simulink model "estimator_designs_main"  (R2022b)
settings: Solver=ode4  StartTime=0.0  StopTime=T  FixedStep=0.002  RelTol=1e-3
values from neighbouring files (symbols this model uses):
  c_lat_f = u(11)    [modelBasedSpeedEstForKalman.m]    (also in validation.m = 140000)
  c_lat_r = u(12)    [modelBasedSpeedEstForKalman.m]    (also in validation.m = 150000)
  c_lon_f = u(9)    [modelBasedSpeedEstForKalman.m]    (also in validation.m = 180000)
  c_lon_r = u(10)    [modelBasedSpeedEstForKalman.m]    (also in validation.m = 200000)
  dt = u(4)    [kinematicVelocity.m]    (also in modelBasedSpeedEstForKalman.m = u(27); validation.m = 0.01)
  eps_bw_acc = 0.1    [validation.m]
  eps_ekf_m_bw_v_u = 0.5    [validation.m]
  eps_m_v = 1    [validation.m]
  m = u(7)    [modelBasedSpeedEstForKalman.m]    (also in validation.m = 3020)
  num_of_signals = 12    [validation.m]
  P0 = diag([1e-5, 1e-5, 1e-5])    [validation.m]
  Q_ekf_1 = diag([1e-5, 1e-2, 1e-2])    [validation.m]
  R = u(9)    [bestWheelSpeedUpdate.m]    (also in modelBasedSpeedEstForKalman.m = u(13); validation.m = 0.3615)
  r_COG_FL = u(10:12)    [bestWheelSpeedUpdate.m]    (also in validation.m = [wheelbase_COG_front; front_track_width / 2; 0])
  r_COG_FR = u(13:15)    [bestWheelSpeedUpdate.m]    (also in validation.m = [wheelbase_COG_front; -front_track_width / 2; 0])
  r_COG_RL = u(16:18)    [bestWheelSpeedUpdate.m]    (also in validation.m = [-wheelbase_COG_rear; rear_track_width / 2; 0])
  r_COG_RR = u(19:21)    [bestWheelSpeedUpdate.m]    (also in validation.m = [-wheelbase_COG_rear; -rear_track_width / 2; 0])
  R_ekf_1 = 1e-2    (= 0.01)    [validation.m]
  sequence_length = 50    [validation.m]
  theta_z = 7145    [validation.m]
  thr_ekf_m_bw_v_u = 5    [validation.m]
  x0 = [0.0001; 0.0001; 0.0001]    [validation.m]
undefined symbols (not defined in the file or in its folder): Discrete, Time
libraries: deeplib x2, ctrlSharedLib x1
(part 2 of 2)

== matlab function estimator_designs_main/v_u_estimators/ekf_model_bw/ekf_custom/ekf_model ==
  data: x_in input; P_in input; z_in input; Q_in input; R_in input; u_in input; fdStep input; x_out output; gateNIS input; P_out output; K_out output; nu_out output; S_out output; x_pred_out output; P_pred_out output; z_pred_out output; F_out output; H_out output; NIS_out output; status_out output
function [x_out,P_out,K_out,nu_out,S_out, ...
          x_pred_out,P_pred_out,z_pred_out, ...
          F_out,H_out,NIS_out,status_out] = ...
    ekf_modelBased_textbook_step(x_in,P_in,z_in,Q_in,R_in,u_in,fdStep,gateNIS)
% -------------------------------------------------------------------------
% Textbook EKF (single step) for state x = [v_x; v_y; w_z].
% Hard-coded:
%   Process model:    x_pred = modelBasedSpeedEstForKalman(x_in, u_in)
%   Measurement:      z = simpleMeasUpdate(x, u) = x(1)  (longitudinal speed)
%
% Inputs:
%   x_in    : 3x1 prior state estimate (k|k)
%   P_in    : 3x3 prior covariance     (k|k)
%   z_in    : scalar measurement (v_x at time k+1)
%   Q_in    : 3x3 process noise covariance (per step)
%   R_in    : scalar measurement variance
%   u_in    : NUx1 input vector for modelBasedSpeedEstForKalman (fixed size; fill ALL entries)
%   fdStep  : finite-difference step for Jacobian (e.g. 1e-5)
%   gateNIS : gating threshold (Inf to disable; e.g. 6.63 for 99% scalar)
%
% Outputs:
%   x_out       : 3x1 posterior state (k+1|k+1)
%   P_out       : 3x3 posterior covariance
%   K_out       : 3x1 Kalman gain
%   nu_out      : innovation (z - z_pred)
%   S_out       : innovation variance
%   x_pred_out  : 3x1 predicted state (k+1|k)
%   P_pred_out  : 3x3 predicted covariance
%   z_pred_out  : scalar predicted measurement
%   F_out       : 3x3 process Jacobian (finite difference)
%   H_out       : 1x3 measurement Jacobian ([1 0 0])
%   NIS_out     : normalized innovation squared (nu^2 / S)
%   status_out  : diagnostic code:
%                 0 OK
%                 1 Process model produced NaN/Inf
%                 2 FD Jacobian produced NaN/Inf (fallback F=I)
%                 3 Innovation variance invalid (S<=0 -> jittered)
%                 4 Update gated (NIS > gateNIS)
%
% Textbook equations:
%   Predict:  x^- = f(x,u);  P^- = F P F' + Q
%   z^- = h(x^-); nu = z - z^-
%   S  = H P^- H' + R
%   K  = P^- H' / S
%   x  = x^- + K nu
%   P  = (I - K H) P^- (I - K H)' + K R K'
%
% -------------------------------------------------------------------------

% ---------- Initialize outputs for safety ----------
x_out       = x_in;
P_out       = P_in;
K_out       = zeros(3,1);
nu_out      = 0;
S_out       = 1;
x_pred_out  = x_in;
P_pred_out  = P_in;
z_pred_out  = x_in(1);
F_out       = eye(3);
H_out       = [1 0 0];
NIS_out     = 0;
status_out  = 0;   % assume OK

% ---------- 1. Prediction ----------
x_pred = modelBasedSpeedEstForKalman(x_in, u_in);
if any(~isfinite(x_pred))
    status_out = 1;  % process model failure
    return;
end

% ---------- 2. Finite-difference Jacobian F = df/dx ----------
h = fdStep;
F = zeros(3,3);

% Column 1
xp = x_in; xm = x_in;
xp(1) = xp(1) + h; xm(1) = xm(1) - h;
fp = modelBasedSpeedEstForKalman(xp, u_in);
fm = modelBasedSpeedEstForKalman(xm, u_in);
if any(~isfinite(fp)) || any(~isfinite(fm))
    status_out = 2;
    F = eye(3);
else
    F(:,1) = (fp - fm)/(2*h);
end

% Column 2
xp = x_in; xm = x_in;
xp(2) = xp(2) + h; xm(2) = xm(2) - h;
fp = modelBasedSpeedEstForKalman(xp, u_in);
fm = modelBasedSpeedEstForKalman(xm, u_in);
if any(~isfinite(fp)) || any(~isfinite(fm))
    status_out = 2;
    F(:,2) = 0;  % leave existing or zero
else
    F(:,2) = (fp - fm)/(2*h);
end

% Column 3
xp = x_in; xm = x_in;
xp(3) = xp(3) + h; xm(3) = xm(3) - h;
fp = modelBasedSpeedEstForKalman(xp, u_in);
fm = modelBasedSpeedEstForKalman(xm, u_in);
if any(~isfinite(fp)) || any(~isfinite(fm))
    status_out = 2;
    F(:,3) = 0;
else
    F(:,3) = (fp - fm)/(2*h);
end

F_out = F;

% ---------- 3. Covariance prediction ----------
P_pred = F*P_in*F' + Q_in;
if any(~isfinite(P_pred(:)))
    status_out = max(status_out,2);
    P_pred = P_in + Q_in;  % simple fallback
end

% ---------- 4. Measurement prediction h(x)=x(1) ----------
z_pred = x_pred(1);
H = [1 0 0];

% ---------- 5. Innovation ----------
nu = z_in - z_pred;

% ---------- 6. Innovation variance ----------
S = P_pred(1,1) + R_in;
if ~isfinite(S) || S <= 0
    S = max(R_in,1e-9);
    status_out = max(status_out,3);
end

% ---------- 7. Kalman Gain ----------
K = P_pred(:,1) / S;

% ---------- 8. NIS ----------
NIS = (nu*nu)/S;

% ---------- 9. Gating ----------
gated = false;
if NIS > gateNIS
    x_post = x_pred;
    P_post = P_pred;
    K(:)   = 0;
    gated  = true;
    status_out = 4;
else
    % ---------- 10. Update ----------
    x_post = x_pred + K*nu;

    % ---------- 11. Covariance update (Joseph) ----------
    I = eye(3);
    IKH = I - K*H;
    P_post = IKH * P_pred * IKH' + K*R_in*K';
end

% ---------- 12. Symmetrize ----------
P_post = 0.5*(P_post + P_post');
if any(~isfinite(P_post(:)))
    status_out = max(status_out,3);
    x_post = x_in;
    P_post = P_in;
    K(:) = 0;
end

% ---------- 13. Assign outputs ----------
x_out       = x_post;
P_out       = P_post;
K_out       = K;
nu_out      = nu;
S_out       = S;
x_pred_out  = x_pred;
P_pred_out  = P_pred;
z_pred_out  = z_pred;
H_out       = H;
NIS_out     = NIS;

end

== matlab function estimator_designs_main/meas_inputs/sequence_generator/MATLAB Function1 ==
  data: SENS_IN_ai input; SENS_IN_ai_seq output; SENS_IN_ai_seq_prev input
function SENS_IN_ai_seq = sequence_generator_t(SENS_IN_ai, SENS_IN_ai_seq_prev)
% This function returns a sequence of data that will be fed into the RNN
% model

    SENS_IN_ai_seq = [SENS_IN_ai_seq_prev(:, 2 : end), SENS_IN_ai];

end

== matlab function estimator_designs_main/v_u_estimators/kf_sm_bw/meas_update_bw/best_wheel_speed_est ==
  data: u input size=23; v_u_bw output size=1; sign_acc output size=1
function [v_u_bw, sign_acc]= bestWheelSpeedUpdate(u)

omega_w_FL = u(1);
omega_w_FR = u(2);
omega_w_RL = u(3);
omega_w_RR = u(4);

delta_FL = u(5);
delta_FR = u(5);
delta_RL = u(6);
delta_RR = u(6);

w_z = u(7);

acc = u(8);

R = u(9);
r_COG_FL = u(10:12);
r_COG_FR = u(13:15);
r_COG_RL = u(16:18);
r_COG_RR = u(19:21);

eps_bw_acc = u(22);

prev_sign_acc = u(23);

w = [0; 0; w_z];

% calculating the velocities of the wheels from the wheel rotational speeds
v_w_FL = [omega_w_FL * R; 0; 0];
v_w_FR = [omega_w_FR * R; 0; 0];
v_w_RL = [omega_w_RL * R; 0; 0];
v_w_RR = [omega_w_RR * R; 0; 0];

% transforming the wheel velocities to the coordinate system in the wheels
% parallel to the one in COG
T_FL = [cos(-delta_FL), sin(-delta_FL), 0; -sin(-delta_FL), cos(-delta_FL), 0; 0, 0, 1];
T_FR = [cos(-delta_FR), sin(-delta_FR), 0; -sin(-delta_FR), cos(-delta_FR), 0; 0, 0, 1];
T_RL = [cos(-delta_RL), sin(-delta_RL), 0; -sin(-delta_RL), cos(-delta_RL), 0; 0, 0, 1];
T_RR = [cos(-delta_RR), sin(-delta_RR), 0; -sin(-delta_RR), cos(-delta_RR), 0; 0, 0, 1];

v_w_FL_T = T_FL * v_w_FL;
v_w_FR_T = T_FR * v_w_FR;
v_w_RL_T = T_RL * v_w_RL;
v_w_RR_T = T_RR * v_w_RR;

% transforming the velocities to COG
v_COG_FL = v_w_FL_T + cross(w, r_COG_FL);
v_COG_FR = v_w_FR_T + cross(w, r_COG_FR);
v_COG_RL = v_w_RL_T + cross(w, r_COG_RL);
v_COG_RR = v_w_RR_T + cross(w, r_COG_RR);

% choosing the best wheel

veh_COG_u = [v_COG_FL(1), v_COG_FR(1), v_COG_RL(1), v_COG_RR(1)];

if abs(acc) < eps_bw_acc
    sign_acc = prev_sign_acc;
else
    sign_acc = sign(acc);
end

if sign_acc <= 0
    v_u_bw = max(veh_COG_u);
else
    v_u_bw = min(veh_COG_u);
end

end

== matlab function estimator_designs_main/v_u_estimators/kf_sm_bw/meas_update_ai/runONNXInference1 ==
  data: inputs input; speed_values output
function speed_values = runONNXInference(inputs)
%#codegen

    coder.extrinsic('run_inference');

    % Preallocate output with fixed size
    speed_values = zeros(1, 1, 'double');

    % Call Python inference function
    temp = run_inference(inputs);

    % Assign result to output
    speed_values = temp;

end

== matlab function estimator_designs_main/v_u_estimators/ekf_model_bw/ekf_custom/MATLAB Function2 ==
  data: x_hat input; Q_cov output size=[3,3]; eps_u input; v_u_threshold input; Q_cov_prev input
function Q_cov  = timeVaryingQ(x_hat, eps_u, v_u_threshold, Q_cov_prev)

v_u_low = v_u_threshold - eps_u;
v_u_up = v_u_threshold + eps_u;

if x_hat(1) < v_u_low
    Q_cov = diag([1e5, 0.1, 0.1]);
    
elseif x_hat(1) > v_u_up
    Q_cov = diag([0.1, 0.1, 0.1]);
else
    Q_cov = Q_cov_prev;    
end

end

== matlab function estimator_designs_main/v_u_estimators/ekf_model_bw/ekf_custom/MATLAB Function1 ==
  data: R_cov_prev input; eps_u input; v_u_threshold input; x_hat input; R_cov output
function R_cov = timeVaryingR(R_cov_prev, eps_u, v_u_threshold, x_hat)

v_u_low = v_u_threshold - eps_u;
v_u_up = v_u_threshold + eps_u;

if x_hat(1) < v_u_low
    R_cov = 1e-5;

elseif x_hat(1) > v_u_up
    R_cov = 1e6;
else
    R_cov = R_cov_prev;
end

if x_hat(2) > 0.5
    R_cov = 1e5;
end

end

== matlab function estimator_designs_main/v_u_estimators/ekf_model_ai/ai_inference_function/runONNXInference1 ==
  data: inputs input; speed_values output
function speed_values = runONNXInference(inputs)
%#codegen

    coder.extrinsic('run_inference');

    % Preallocate output with fixed size
    speed_values = zeros(1, 1, 'double');

    % Call Python inference function
    temp = run_inference(inputs);

    % Assign result to output
    speed_values = temp;

end

== matlab function estimator_designs_main/v_u_estimators/best_wheel/best_wheel_speed_est ==
  data: u input size=23; v_u_bw output size=1; sign_acc output size=1
function [v_u_bw, sign_acc]= bestWheelSpeedUpdate(u)

omega_w_FL = u(1);
omega_w_FR = u(2);
omega_w_RL = u(3);
omega_w_RR = u(4);

delta_FL = u(5);
delta_FR = u(5);
delta_RL = u(6);
delta_RR = u(6);

w_z = u(7);

acc = u(8);

R = u(9);
r_COG_FL = u(10:12);
r_COG_FR = u(13:15);
r_COG_RL = u(16:18);
r_COG_RR = u(19:21);

eps_bw_acc = u(22);

prev_sign_acc = u(23);

w = [0; 0; w_z];

% calculating the velocities of the wheels from the wheel rotational speeds
v_w_FL = [omega_w_FL * R; 0; 0];
v_w_FR = [omega_w_FR * R; 0; 0];
v_w_RL = [omega_w_RL * R; 0; 0];
v_w_RR = [omega_w_RR * R; 0; 0];

% transforming the wheel velocities to the coordinate system in the wheels
% parallel to the one in COG
T_FL = [cos(-delta_FL), sin(-delta_FL), 0; -sin(-delta_FL), cos(-delta_FL), 0; 0, 0, 1];
T_FR = [cos(-delta_FR), sin(-delta_FR), 0; -sin(-delta_FR), cos(-delta_FR), 0; 0, 0, 1];
T_RL = [cos(-delta_RL), sin(-delta_RL), 0; -sin(-delta_RL), cos(-delta_RL), 0; 0, 0, 1];
T_RR = [cos(-delta_RR), sin(-delta_RR), 0; -sin(-delta_RR), cos(-delta_RR), 0; 0, 0, 1];

v_w_FL_T = T_FL * v_w_FL;
v_w_FR_T = T_FR * v_w_FR;
v_w_RL_T = T_RL * v_w_RL;
v_w_RR_T = T_RR * v_w_RR;

% transforming the velocities to COG
v_COG_FL = v_w_FL_T + cross(w, r_COG_FL);
v_COG_FR = v_w_FR_T + cross(w, r_COG_FR);
v_COG_RL = v_w_RL_T + cross(w, r_COG_RL);
v_COG_RR = v_w_RR_T + cross(w, r_COG_RR);

% choosing the best wheel

veh_COG_u = [v_COG_FL(1), v_COG_FR(1), v_COG_RL(1), v_COG_RR(1)];

if abs(acc) < eps_bw_acc
    sign_acc = prev_sign_acc;
else
    sign_acc = sign(acc);
end

if sign_acc <= 0
    v_u_bw = max(veh_COG_u);
else
    v_u_bw = min(veh_COG_u);
end

end

== matlab function estimator_designs_main/v_u_estimators/ekf_model_ai/ekf_custom/MATLAB Function1 ==
  data: R_cov_prev input; eps_u input; v_u_threshold input; x_hat input; R_cov output
function R_cov = timeVaryingR(R_cov_prev, eps_u, v_u_threshold, x_hat)

v_u_low = v_u_threshold - eps_u;
v_u_up = v_u_threshold + eps_u;

if x_hat(1) < v_u_low
    R_cov = 0.0001;

elseif x_hat(1) > v_u_up
    R_cov = 0.01;
else
    R_cov = R_cov_prev;
end


end

== matlab function estimator_designs_main/meas_inputs/sequence_generator/MATLAB Function4 ==
  data: SNES_IN_ai input; SENS_IN_ai_seq output; SENS_IN_ai_seq_prev input
function SENS_IN_ai_seq = sequence_generator_inf(SNES_IN_ai, SENS_IN_ai_seq_prev)
% This function returns a sequence of data that will be fed into the RNN
% model

    SENS_IN_ai_seq = [SENS_IN_ai_seq_prev(2 : end, :); SNES_IN_ai'];

end

== matlab function estimator_designs_main/v_u_estimators/ekf_model_bw/meas_update_bw/best_wheel_speed_est ==
  data: u input size=23; v_u_bw output size=1; sign_acc output size=1
function [v_u_bw, sign_acc]= bestWheelSpeedUpdate(u)

omega_w_FL = u(1);
omega_w_FR = u(2);
omega_w_RL = u(3);
omega_w_RR = u(4);

delta_FL = u(5);
delta_FR = u(5);
delta_RL = u(6);
delta_RR = u(6);

w_z = u(7);

acc = u(8);

R = u(9);
r_COG_FL = u(10:12);
r_COG_FR = u(13:15);
r_COG_RL = u(16:18);
r_COG_RR = u(19:21);

eps_bw_acc = u(22);

prev_sign_acc = u(23);

w = [0; 0; w_z];

% calculating the velocities of the wheels from the wheel rotational speeds
v_w_FL = [omega_w_FL * R; 0; 0];
v_w_FR = [omega_w_FR * R; 0; 0];
v_w_RL = [omega_w_RL * R; 0; 0];
v_w_RR = [omega_w_RR * R; 0; 0];

% transforming the wheel velocities to the coordinate system in the wheels
% parallel to the one in COG
T_FL = [cos(-delta_FL), sin(-delta_FL), 0; -sin(-delta_FL), cos(-delta_FL), 0; 0, 0, 1];
T_FR = [cos(-delta_FR), sin(-delta_FR), 0; -sin(-delta_FR), cos(-delta_FR), 0; 0, 0, 1];
T_RL = [cos(-delta_RL), sin(-delta_RL), 0; -sin(-delta_RL), cos(-delta_RL), 0; 0, 0, 1];
T_RR = [cos(-delta_RR), sin(-delta_RR), 0; -sin(-delta_RR), cos(-delta_RR), 0; 0, 0, 1];

v_w_FL_T = T_FL * v_w_FL;
v_w_FR_T = T_FR * v_w_FR;
v_w_RL_T = T_RL * v_w_RL;
v_w_RR_T = T_RR * v_w_RR;

% transforming the velocities to COG
v_COG_FL = v_w_FL_T + cross(w, r_COG_FL);
v_COG_FR = v_w_FR_T + cross(w, r_COG_FR);
v_COG_RL = v_w_RL_T + cross(w, r_COG_RL);
v_COG_RR = v_w_RR_T + cross(w, r_COG_RR);

% choosing the best wheel

veh_COG_u = [v_COG_FL(1), v_COG_FR(1), v_COG_RL(1), v_COG_RR(1)];

if abs(acc) < eps_bw_acc
    sign_acc = prev_sign_acc;
else
    sign_acc = sign(acc);
end

if sign_acc <= 0
    v_u_bw = max(veh_COG_u);
else
    v_u_bw = min(veh_COG_u);
end

end

== matlab function estimator_designs_main/v_u_estimators/ekf_model_ai/ekf_custom/MATLAB Function2 ==
  data: x_hat input; Q_cov output size=[3,3]; eps_u input; v_u_threshold input; Q_cov_prev input
function Q_cov  = timeVaryingQ(x_hat, eps_u, v_u_threshold, Q_cov_prev)

v_u_low = v_u_threshold - eps_u;
v_u_up = v_u_threshold + eps_u;

if x_hat(1) < v_u_low
    Q_cov = diag([100, 0.001, 0.001]);
    
elseif x_hat(1) > v_u_up
    Q_cov = diag([0.01, 0.001, 0.001]);
else
    Q_cov = Q_cov_prev;    
end

end

== matlab function estimator_designs_main/v_u_estimators/ekf_model_ai/ekf_custom/ekf_model ==
  data: x_in input; P_in input; z_in input; Q_in input; R_in input; u_in input; fdStep input; x_out output; gateNIS input; P_out output; K_out output; nu_out output; S_out output; x_pred_out output; P_pred_out output; z_pred_out output; F_out output; H_out output; NIS_out output; status_out output
function [x_out,P_out,K_out,nu_out,S_out, ...
          x_pred_out,P_pred_out,z_pred_out, ...
          F_out,H_out,NIS_out,status_out] = ...
    ekf_modelBased_textbook_step(x_in,P_in,z_in,Q_in,R_in,u_in,fdStep,gateNIS)
% -------------------------------------------------------------------------
% Textbook EKF (single step) for state x = [v_x; v_y; w_z].
% Hard-coded:
%   Process model:    x_pred = modelBasedSpeedEstForKalman(x_in, u_in)
%   Measurement:      z = simpleMeasUpdate(x, u) = x(1)  (longitudinal speed)
%
% Inputs:
%   x_in    : 3x1 prior state estimate (k|k)
%   P_in    : 3x3 prior covariance     (k|k)
%   z_in    : scalar measurement (v_x at time k+1)
%   Q_in    : 3x3 process noise covariance (per step)
%   R_in    : scalar measurement variance
%   u_in    : NUx1 input vector for modelBasedSpeedEstForKalman (fixed size; fill ALL entries)
%   fdStep  : finite-difference step for Jacobian (e.g. 1e-5)
%   gateNIS : gating threshold (Inf to disable; e.g. 6.63 for 99% scalar)
%
% Outputs:
%   x_out       : 3x1 posterior state (k+1|k+1)
%   P_out       : 3x3 posterior covariance
%   K_out       : 3x1 Kalman gain
%   nu_out      : innovation (z - z_pred)
%   S_out       : innovation variance
%   x_pred_out  : 3x1 predicted state (k+1|k)
%   P_pred_out  : 3x3 predicted covariance
%   z_pred_out  : scalar predicted measurement
%   F_out       : 3x3 process Jacobian (finite difference)
%   H_out       : 1x3 measurement Jacobian ([1 0 0])
%   NIS_out     : normalized innovation squared (nu^2 / S)
%   status_out  : diagnostic code:
%                 0 OK
%                 1 Process model produced NaN/Inf
%                 2 FD Jacobian produced NaN/Inf (fallback F=I)
%                 3 Innovation variance invalid (S<=0 -> jittered)
%                 4 Update gated (NIS > gateNIS)
%
% Textbook equations:
%   Predict:  x^- = f(x,u);  P^- = F P F' + Q
%   z^- = h(x^-); nu = z - z^-
%   S  = H P^- H' + R
%   K  = P^- H' / S
%   x  = x^- + K nu
%   P  = (I - K H) P^- (I - K H)' + K R K'
%
% -------------------------------------------------------------------------

% ---------- Initialize outputs for safety ----------
x_out       = x_in;
P_out       = P_in;
K_out       = zeros(3,1);
nu_out      = 0;
S_out       = 1;
x_pred_out  = x_in;
P_pred_out  = P_in;
z_pred_out  = x_in(1);
F_out       = eye(3);
H_out       = [1 0 0];
NIS_out     = 0;
status_out  = 0;   % assume OK

% ---------- 1. Prediction ----------
x_pred = modelBasedSpeedEstForKalman(x_in, u_in);
if any(~isfinite(x_pred))
    status_out = 1;  % process model failure
    return;
end

% ---------- 2. Finite-difference Jacobian F = df/dx ----------
h = fdStep;
F = zeros(3,3);

% Column 1
xp = x_in; xm = x_in;
xp(1) = xp(1) + h; xm(1) = xm(1) - h;
fp = modelBasedSpeedEstForKalman(xp, u_in);
fm = modelBasedSpeedEstForKalman(xm, u_in);
if any(~isfinite(fp)) || any(~isfinite(fm))
    status_out = 2;
    F = eye(3);
else
    F(:,1) = (fp - fm)/(2*h);
end

% Column 2
xp = x_in; xm = x_in;
xp(2) = xp(2) + h; xm(2) = xm(2) - h;
fp = modelBasedSpeedEstForKalman(xp, u_in);
fm = modelBasedSpeedEstForKalman(xm, u_in);
if any(~isfinite(fp)) || any(~isfinite(fm))
    status_out = 2;
    F(:,2) = 0;  % leave existing or zero
else
    F(:,2) = (fp - fm)/(2*h);
end

% Column 3
xp = x_in; xm = x_in;
xp(3) = xp(3) + h; xm(3) = xm(3) - h;
fp = modelBasedSpeedEstForKalman(xp, u_in);
fm = modelBasedSpeedEstForKalman(xm, u_in);
if any(~isfinite(fp)) || any(~isfinite(fm))
    status_out = 2;
    F(:,3) = 0;
else
    F(:,3) = (fp - fm)/(2*h);
end

F_out = F;

% ---------- 3. Covariance prediction ----------
P_pred = F*P_in*F' + Q_in;
if any(~isfinite(P_pred(:)))
    status_out = max(status_out,2);
    P_pred = P_in + Q_in;  % simple fallback
end

% ---------- 4. Measurement prediction h(x)=x(1) ----------
z_pred = x_pred(1);
H = [1 0 0];

% ---------- 5. Innovation ----------
nu = z_in - z_pred;

% ---------- 6. Innovation variance ----------
S = P_pred(1,1) + R_in;
if ~isfinite(S) || S <= 0
    S = max(R_in,1e-9);
    status_out = max(status_out,3);
end

% ---------- 7. Kalman Gain ----------
K = P_pred(:,1) / S;

% ---------- 8. NIS ----------
NIS = (nu*nu)/S;

% ---------- 9. Gating ----------
gated = false;
if NIS > gateNIS
    x_post = x_pred;
    P_post = P_pred;
    K(:)   = 0;
    gated  = true;
    status_out = 4;
else
    % ---------- 10. Update ----------
    x_post = x_pred + K*nu;

    % ---------- 11. Covariance update (Joseph) ----------
    I = eye(3);
    IKH = I - K*H;
    P_post = IKH * P_pred * IKH' + K*R_in*K';
end

% ---------- 12. Symmetrize ----------
P_post = 0.5*(P_post + P_post');
if any(~isfinite(P_post(:)))
    status_out = max(status_out,3);
    x_post = x_in;
    P_post = P_in;
    K(:) = 0;
end

% ---------- 13. Assign outputs ----------
x_out       = x_post;
P_out       = P_post;
K_out       = K;
nu_out      = nu;
S_out       = S;
x_pred_out  = x_pred;
P_pred_out  = P_pred;
z_pred_out  = z_pred;
H_out       = H;
NIS_out     = NIS;

end
